simulink model "myTwoInTowOne"  (R2024a)
settings: Solver=VariableStepAuto  StartTime=0.0  StopTime=10.0  RelTol=1e-3
InitFcn:
  | close all;
  | clear all;
  | % Excelファイルのパスとファイル名
  | [file, path] = uigetfile('*.xlsx', 'Excelファイルを選択してください');
  | if isequal(file, 0)
  |     disp('ファイルが選択されませんでした。');
  |     return;
  | else
  |     filepath = fullfile(path, file);
  | end
  | % シート名またはシートインデックス
  | sheet = 'Sheet1'; % シート名を指定する場合
  | % sheet = 1; % シートインデックスを指定する場合
  | % Excelファイルからデータを読み込む
  | data = readcell(filepath, 'Sheet', sheet);
  | x1 = cellfun(@double, data(2:end, 1));
  | x2 = cellfun(@double, data(2:end, 2));
StopFcn:
  | y = out.y.Data;
  | figure;
  | scatter(x1(y == -1), x2(y == -1), 'filled', 'b'); % yが0の点をでプロット
  | hold on
  | scatter(x1(y == 1), x2(y == 1), 'filled', 'r'); % yが1の点を赤でプロット
  | grid on
settings Model: Creator=mashi  LastModifiedBy=mashi

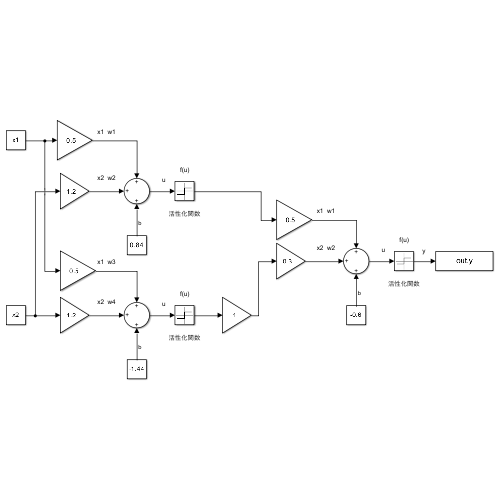
[thumbnail: Simulink's stored preview of the top-level diagram]
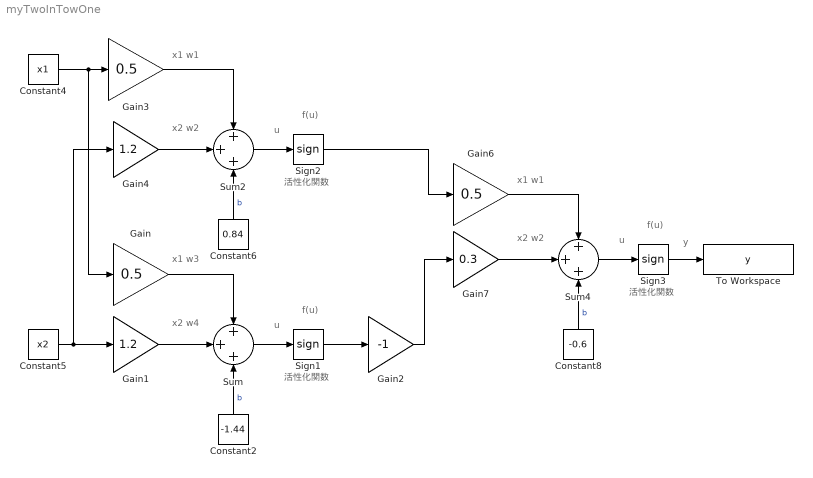
== system myTwoInTowOne ==
  note: y
  note: 活性化関数
  note: u
  note: f(u)
  note: x2 w4
  note: x1 w3
  note: 活性化関数
  note: u
  note: f(u)
  note: x2 w2
  note: x1 w1
  note: 活性化関数
  note: u
  note: f(u)
  note: x2 w2
  note: x1 w1
  Constant2 : Constant  Value=-1.44
  Constant4 : Constant  Value=x1
  Constant5 : Constant  Value=x2
  Constant6 : Constant  Value=0.84
  Constant8 : Constant  Value=-0.6
  Gain : Gain  Gain=0.5
  Gain1 : Gain  Gain=1.2
  Gain2 : Gain  Gain=-1
  Gain3 : Gain  Gain=0.5
  Gain4 : Gain  Gain=1.2
  Gain6 : Gain  Gain=0.5
  Gain7 : Gain  Gain=0.3
  Sign1 : Signum
  Sign2 : Signum
  Sign3 : Signum
  Sum : Sum  Inputs=+++
  Sum2 : Sum  Inputs=+++
  Sum4 : Sum  Inputs=+++
  To Workspace : ToWorkspace  VariableName=y  SaveFormat=Timeseries  SampleTime=-1
  wires:
  Gain/1 -> Sum/1
  Gain1/1 -> Sum/2
  Sum/1 -> Sign1/1
  Constant2/1 -> Sum/3  "b"
  Constant6/1 -> Sum2/3  "b"
  Sum2/1 -> Sign2/1
  Gain4/1 -> Sum2/2
  Gain3/1 -> Sum2/1
  Constant4/1 -> Gain/1, Gain3/1
  Constant8/1 -> Sum4/3  "b"
  Sum4/1 -> Sign3/1
  Gain7/1 -> Sum4/2
  Gain6/1 -> Sum4/1
  Constant5/1 -> Gain4/1, Gain1/1
  Sign2/1 -> Gain6/1
  Sign1/1 -> Gain2/1
  Sign3/1 -> To Workspace/1
  Gain2/1 -> Gain7/1
